simulink model "sinal_de_controle_robustez"  (R2015a)
settings: Solver=ode23t  StartTime=0.0  StopTime=10.0  RelTol=1e-3
values from neighbouring files (symbols this model uses):
  Bs = 7.5    [espaco_estados.m]    (also in modelagem_Suspensao_Ativa.m; modelagem_atualizada.m; teste_de_robustez_EE.m = linspace(6.75, 8.25, 7))
  K1 = place(A,B,polos2)    [alocacao_dos_polos.m]    (also in teste_de_robustez_EE.m = 24.66)
  K2 = 48.87    [teste_de_robustez_EE.m]
  K3 = -0.47    [teste_de_robustez_EE.m]
  K4 = 3.68    [teste_de_robustez_EE.m]
  Ks = 900    [espaco_estados.m]    (also in modelagem_Suspensao_Ativa.m; modelagem_atualizada.m; teste_de_robustez_EE.m = linspace(900-(900*0.05), 900+(900*0.05), 7))
  Kus = 1250    [espaco_estados.m]    (also in modelagem_Suspensao_Ativa.m; modelagem_atualizada.m; teste_de_robustez_EE.m = linspace(1250-(1250*0.05), 1250+(1250*0.05), 7))
  Ms = 2.45    [espaco_estados.m]    (also in modelagem_Suspensao_Ativa.m; modelagem_atualizada.m; teste_de_robustez_EE.m)
  Mus = 1    [espaco_estados.m]    (also in modelagem_Suspensao_Ativa.m; modelagem_atualizada.m; teste_de_robustez_EE.m)
undefined symbols (not defined in the file or in its folder): bs, bus, ks, kus
settings Model: Creator=Joacy Mesquita  LastModifiedBy=Joacy Mesquita

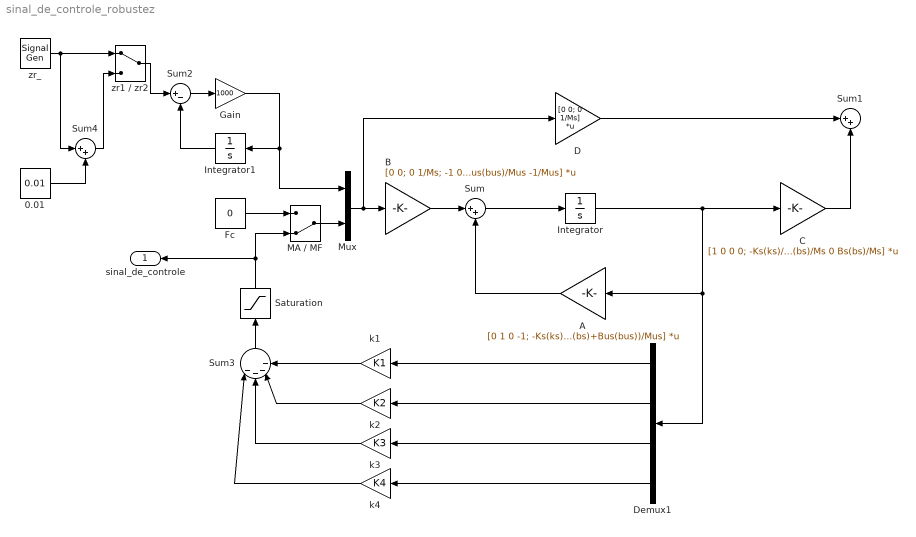
== system sinal_de_controle_robustez ==
  0.01 : Constant  Value=0.01
  A : Gain  Gain=[0 1 0 -1; -Ks(ks)/Ms -Bs(bs)/Ms 0 Bs(bs)/Ms; 0 0 0 1; Ks(ks)/Mus Bs(bs)/Mus -Kus(kus)/Mus -(Bs(bs)+Bus(bus))/Mus]  Multiplication=Matrix(K*u)
  B : Gain  Gain=[0 0; 0 1/Ms; -1 0; Bus(bus)/Mus -1/Mus]  Multiplication=Matrix(K*u)
  C : Gain  Gain=[1 0 0 0; -Ks(ks)/Ms -Bs(bs)/Ms 0 Bs(bs)/Ms]  Multiplication=Matrix(K*u)
  D : Gain  Gain=[0 0; 0 1/Ms]  Multiplication=Matrix(K*u)
  Demux1 : Demux
  Fc : Constant  Value=0
  Gain : Gain  Gain=1000
  Integrator : Integrator
  Integrator1 : Integrator
  MA / MF : ManualSwitch  CurrentSetting=0
  Mux : Mux  Inputs=2
  Saturation : Saturate  UpperLimit=30  LowerLimit=-30
  Sum : Sum  Inputs=|++
  Sum1 : Sum  Inputs=|++
  Sum2 : Sum  Inputs=|+-
  Sum3 : Sum  Inputs=|----
  Sum4 : Sum  Inputs=|++
  k1 : Gain  Gain=K1
  k2 : Gain  Gain=K2
  k3 : Gain  Gain=K3
  k4 : Gain  Gain=K4
  zr1 / zr2 : ManualSwitch
  zr_ : SignalGenerator  WaveForm=square  Amplitude=-0.01  Frequency=0.3
  sinal_de_controle : Outport
  wires:
  Mux/1 -> B/1, D/1
  B/1 -> Sum/1
  Sum/1 -> Integrator/1
  Integrator/1 -> C/1, Demux1/1, A/1
  D/1 -> Sum1/1
  C/1 -> Sum1/2
  zr_/1 -> zr1 / zr2/1, Sum4/1
  Gain/1 -> Integrator1/1, Mux/1
  Sum2/1 -> Gain/1
  Integrator1/1 -> Sum2/2
  Demux1/1 -> k1/1
  Demux1/2 -> k2/1
  Demux1/3 -> k3/1
  MA / MF/1 -> Mux/2
  Fc/1 -> MA / MF/1
  k1/1 -> Sum3/4
  k2/1 -> Sum3/3
  k3/1 -> Sum3/2
  Sum3/1 -> Saturation/1
  A/1 -> Sum/2
  Demux1/4 -> k4/1
  Saturation/1 -> MA / MF/2, sinal_de_controle/1
  k4/1 -> Sum3/1
  Sum4/1 -> zr1 / zr2/2
  0.01/1 -> Sum4/2
  zr1 / zr2/1 -> Sum2/1
